simulink model "ACDCACsummarycircuit"  (R2023b)
settings: Solver=ode8  StartTime=0.0  StopTime=1  FixedStep=1e-7  MaxStep=1e-8  RelTol=1e-3
libraries: spsMosfetLib x6, spsSeriesRLCBranchLib x5, spsVoltageMeasurementLib x3, spsCurrentMeasurementLib x2, spsIGBTDiodeLib x2, powerlib_extras x2, spsTHDLib x2, simulink x2, spsACVoltageSourceLib x1, spsMeanLib x1, slpidlib x1, spsPLLLib x1
settings Model: SimulationMode=accelerator  Creator=LENOVO  LastModifiedBy=45276
settings SolverCC: ZeroCrossAlgorithm=Adaptive
settings DebuggingCC: MaskedZcDiagnostic=none  IgnoredZcDiagnostic=none

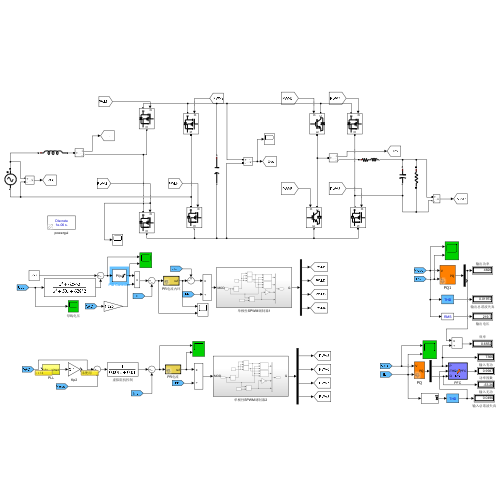
[thumbnail: Simulink's stored preview of the top-level diagram]
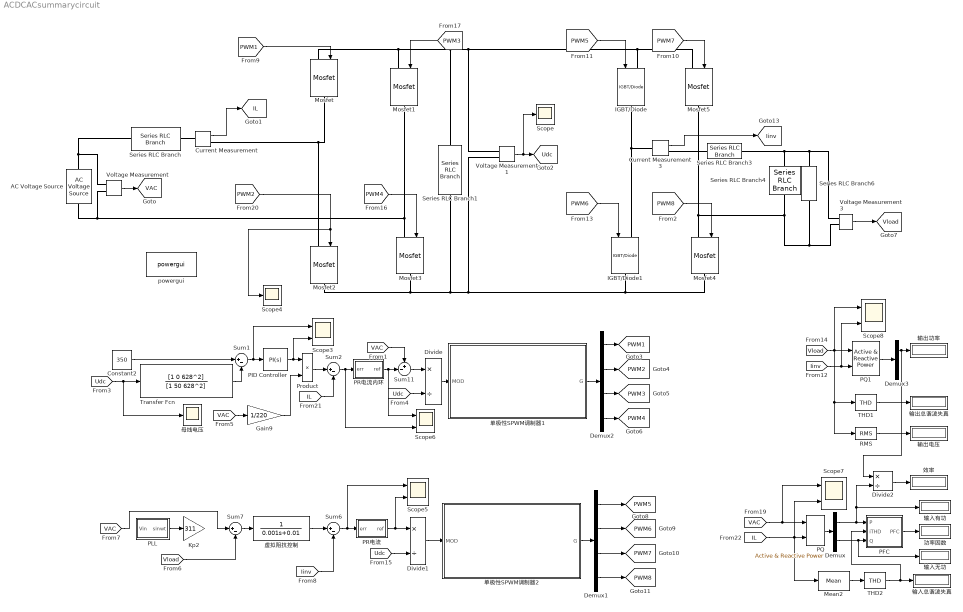
== system ACDCACsummarycircuit ==
  AC Voltage Source : spsACVoltageSourceLib/AC Voltage Source  Amplitude=311  Phase=0  Frequency=50  SampleTime=0  Measurements=None  BusType=swing  Pref=10e3  Qref=0  Qmin=-inf  Qmax=+inf
  Constant2 : Constant  Value=350
  Current Measurement : spsCurrentMeasurementLib/Current Measurement  PhasorSimulation=off  OutputType=Complex  PSBequivalent=0
  Current Measurement3 : spsCurrentMeasurementLib/Current Measurement  PhasorSimulation=off  OutputType=Complex  PSBequivalent=0
  Demux : Demux  Outputs=2
  Demux1 : Demux
  Demux2 : Demux
  Demux3 : Demux  Outputs=2
  Divide : Product  Inputs=*/
  Divide1 : Product  Inputs=*/
  Divide2 : Product  Inputs=*/
  Gain9 : Gain  Gain=1/220
  IGBT/Diode : spsIGBTDiodeLib/IGBT//Diode  Ron=1e-3  Rs=1e5  Cs=inf  Measurements=off
  IGBT/Diode1 : spsIGBTDiodeLib/IGBT//Diode  Ron=1e-3  Rs=1e5  Cs=inf  Measurements=off
  Kp2 : Gain  Gain=311
  Mean2 : spsMeanLib/Mean  Freq=10000  Vinit=0  Ts=0
  Mosfet{,1..5} (6 alike) : spsMosfetLib/Mosfet  Ron=0.05  Lon=0  Rd=0.01  Vfd=1  IC=0  Rs=1e5  Cs=inf  Measurements=off
  PFC : MATLAB Function  TreatAsAtomicUnit=on
  PID Controller : slpidlib/PID Controller  Controller=PI  Form=Parallel  TimeDomain=Continuous-time  UseExternalTs=off  SampleTime=-1  IntegratorMethod=Forward Euler  FilterMethod=Forward Euler  ControllerParametersSource=internal  P=0.4  I=10  UseKiTs=off  D=0.001  N=100  UseFilter=on  TunerSelectOption=Transfer Function Based (PID Tuner App)  InitialConditionSource=internal  InitialConditionForIntegrator=0  InitialConditionForFilter=0  DifferentiatorICPrevScaledInput=0  ExternalReset=none  TrackingMode=off  Kt=1  LimitOutput=on  SatLimitsSource=internal  UpperSaturationLimit=200  LowerSaturationLimit=-200  LinearizeAsGain=on  AntiWindupMode=clamping  Kb=1  LimitIntegrator=off  UpperIntegratorSaturationLimit=inf  LowerIntegratorSaturationLimit=-inf  POutMin=[]  POutMax=[]  IOutMin=[]  IOutMax=[]  DOutMin=[]  DOutMax=[]  NOutMin=[]  NOutMax=[]  SumOutMin=[]  SumOutMax=[]  SaturationOutMin=[]  SaturationOutMax=[]  PParamMin=[]  PParamMax=[]  IParamMin=[]  IParamMax=[]  DParamMin=[]  DParamMax=[]  NParamMin=[]  NParamMax=[]  KbParamMin=[]  KbParamMax=[]  KtParamMin=[]  KtParamMax=[]  KbOutMin=[]  KbOutMax=[]  KtOutMin=[]  KtOutMax=[]  IntegratorOutMin=[]  IntegratorOutMax=[]  FilterOutMin=[]  FilterOutMax=[]  SumI1OutMin=[]  SumI1OutMax=[]  SumI2OutMin=[]  SumI2OutMax=[]  SumI3OutMin=[]  SumI3OutMax=[]  SumI4OutMin=[]  SumI4OutMax=[]  SumDOutMin=[]  SumDOutMax=[]  DifferentiatorOutMin=[]  DifferentiatorOutMax=[]  FilterDiffOutCoefMin=[]  FilterDiffOutCoefMax=[]  ReciprocalOutMin=[]  ReciprocalOutMax=[]  SumDenOutMin=[]  SumDenOutMax=[]  SumNumOutMin=[]  SumNumOutMax=[]  DivideOutMin=[]  DivideOutMax=[]  UdiffTsProdOutMin=[]  UdiffTsProdOutMax=[]  NTsProdOutMin=[]  NTsProdOutMax=[]  UintegralTsProdOutMin=[]  UintegralTsProdOutMax=[]  UngainTsProdOutMin=[]  UngainTsProdOutMax=[]  ClampingZeroOutDataTypeStr=Inherit: Inherit via back propagation  ClampingZeroOutMin=[]  ClampingZeroOutMax=[]  FilterDenConstantOutDataTypeStr=Inherit: Inherit via back propagation  FilterDenConstantOutMin=[]  FilterDenConstantOutMax=[]  PCopyOutDataTypeStr=Inherit: Inherit via back propagation  PCopyOutMin=[]  PCopyOutMax=[]  NCopyOutDataTypeStr=Inherit: Inherit via back propagation  NCopyOutMin=[]  NCopyOutMax=[]  IntegratorContinuousStateAttributes=''  IntegratorStateMustResolveToSignalObject=off  IntegratorRTWStateStorageClass=Auto  FilterContinuousStateAttributes=''  FilterStateMustResolveToSignalObject=off  FilterRTWStateStorageClass=Auto  ParallelPVariant=InternalParameters  IdealPVariant=Disabled  IVariant=InternalParameters  DVariant=Disabled  IntegratorVariant=Continuous  SatVariant=Enabled  AWVariant=ContClampingParallel  PCopyVariant=Disabled  TRVariant=Disabled  FdbkBlocksVariant=Forward  IdealPFdbkVariant=Disabled  SatFdbkVariant=Disabled  DerivativeFilterVariant=Disabled  NVariant=Disabled  NCopyVariant=Disabled_SignalSpec  FilterICVariant=Disabled  IntegratorICVariant=InternalICs  ExternalResetVariant=Disabled  TRSumVariant=Passthrough  SumFdbkVariant=Disabled  SumVariant=Sum_PI  TsampFilterVariant=InternalTs  TsampNgainVariant=Passthrough  TsampIntegralVariant=Disabled_SignalSpec  ExternalSaturationOutDataTypeStr=Inherit: Same as second input
  PLL : Subsystem
  PQ : powerlib_extras/Measurements/Active & Reactive Power  f1=50
  PQ1 : powerlib_extras/Measurements/Active & Reactive Power  f1=50
  PR电流 : Subsystem  TreatAsAtomicUnit=on  mask{Kp=2, Kr=300, Wc=5, Upper=1000, Lower=-1000}
  PR电流内环 : Subsystem  TreatAsAtomicUnit=on  mask{Kp=3, Kr=100, Wc=5, Upper=310, Lower=-310}
  Product : Product
  RMS : spsRMSLib/RMS  TrueRMS=on  Freq=50  RMSInit=200  Ts=0
  Scope : Scope
  Scope{3,5..8} (5 alike) : Scope  NumInputPorts=2
  Scope4 : Scope
  Series RLC Branch : spsSeriesRLCBranchLib/Series RLC Branch  LConnTagsString=__new0  RConnTagsString=__new0  BranchType=L  Resistance=1  Inductance=6e-4  SetiL0=off  InitialCurrent=0  Capacitance=1e-6  Setx0=off  InitialVoltage=0  Measurements=None
  Series RLC Branch1 : spsSeriesRLCBranchLib/Series RLC Branch  LConnTagsString=__new0  RConnTagsString=__new0  BranchType=C  Resistance=1  Inductance=1e-3  SetiL0=off  InitialCurrent=0  Capacitance=4e-3  Setx0=on  InitialVoltage=310  Measurements=None
  Series RLC Branch3 : spsSeriesRLCBranchLib/Series RLC Branch  LConnTagsString=__new0  RConnTagsString=__new0  BranchType=RL  Resistance=0.05  Inductance=1e-3  SetiL0=off  InitialCurrent=0  Capacitance=1e-6  Setx0=off  InitialVoltage=0  Measurements=None
  Series RLC Branch4 : spsSeriesRLCBranchLib/Series RLC Branch  LConnTagsString=__new0  RConnTagsString=__new0  BranchType=C  Resistance=0.0042  Inductance=1e-3  SetiL0=off  InitialCurrent=0  Capacitance=6e-6  Setx0=off  InitialVoltage=0  Measurements=None
  Series RLC Branch6 : spsSeriesRLCBranchLib/Series RLC Branch  LConnTagsString=__new0  RConnTagsString=__new0  BranchType=R  Resistance=10  Inductance=1e-3  SetiL0=off  InitialCurrent=0  Capacitance=1e-4  Setx0=off  InitialVoltage=0  Measurements=None
  Sum{1..2,6..7} (4 alike) : Sum  Inputs=|+-
  Sum11 : Sum  Inputs=+-|
  THD1 : spsTHDLib/THD  Freq=50  Ts=0
  THD2 : spsTHDLib/THD  Freq=50  Ts=0
  Transfer Fcn : TransferFcn  Numerator=[1 0 628^2]  Denominator=[1 50 628^2]
  Voltage Measurement : spsVoltageMeasurementLib/Voltage Measurement  PhasorSimulation=off  OutputType=Complex  PSBequivalent=0
  Voltage Measurement1 : spsVoltageMeasurementLib/Voltage Measurement  PhasorSimulation=off  OutputType=Complex  PSBequivalent=0
  Voltage Measurement3 : spsVoltageMeasurementLib/Voltage Measurement  PhasorSimulation=off  OutputType=Complex  PSBequivalent=0
  powergui : sps_lib/powergui  Priority=1  SimulationMode=Discrete  SampleTime=1e-6  frequency=60  Iterations=50  frequencyindice=50  Pbase=100e6  ErrMax=1e-4  UnitsV=kV  UnitsW=MW  buscounter=0  FunctionMessages=off  echomessages=off  EnableUseOfTLC=off  CurrentSourceSwitches=off  DisableSnubberDevices=off  DisableRonSwitches=off  DisableVfSwitches=off  DisplayEquations=off  AutomaticDiscreteSolvers=off  SolverType=Tustin/Backward Euler (TBE)  Interpol=off  ExternalGateDelay=off  methode=off  Ts=100  x0status=blocks  SPID=on  SwTol=0  HookPort=off  NonlinearTolerance=1e-4  nMaxIteration=100  ContinueOnMaxIteration=off  RestoreLinks=warning  ResistiveCurrentMeasurement=off  Frange=[0:2:500]  Ylog=off  Xlog=on  ShowGrid=off  save=off  variable=ZData  structure=0  ZoomFFT=off  StartTime=0.0  cycles=1  DisplayStyle=1  fundamental=60  FreqAxis=off  MaxFrequency=1000  frequencyindicesteady=1  RmsSteady=1  display=off
  功率因数 : Display
  单极性SPWM调制器1 : Subsystem
  单极性SPWM调制器2 : Subsystem
  效率 : Display
  母线电压 : Scope
  虚拟阻抗控制 : TransferFcn  Numerator=1  Denominator=[0.001 0.01]
  输入总谐波失真 : Display
  输入无功 : Display
  输入有功 : Display
  输出功率 : Display
  输出总谐波失真 : Display
  输出电压 : Display
  tag scope: IL=global, Iinv=global, PWM1=global, PWM2=global, PWM3=global, PWM4=global, PWM5=global, PWM6=global, PWM7=global, PWM8=global, Udc=global, VAC=global, Vload=global
  wires:
  Voltage Measurement3/1 -> [Vload]
  [PWM6] -> IGBT/Diode1/1
  [PWM5] -> IGBT/Diode/1
  Current Measurement3/1 -> [Iinv]
  [PWM1] -> Mosfet/1
  [PWM2] -> Scope4/1, Mosfet2/1
  Voltage Measurement/1 -> [VAC]
  Current Measurement/1 -> [IL]
  Constant2/1 -> Sum1/1
  Sum1/1 -> Scope3/1, PID Controller/1
  Gain9/1 -> Product/2
  PID Controller/1 -> Scope3/2, Product/1
  Product/1 -> Sum2/1
  Transfer Fcn/1 -> Sum1/2
  Sum2/1 -> Scope6/2, PR电流内环/1(err)
  [IL] -> Sum2/2
  [Udc] -> Transfer Fcn/1, 母线电压/1
  PR电流内环/1(ref) -> Scope6/1, Sum11/2
  [VAC] -> Sum11/1
  Sum11/1 -> Divide/1
  [Udc] -> Divide/2
  [VAC] -> Gain9/1
  Demux2/1 -> [PWM1]
  Demux2/2 -> [PWM2]
  Sum7/1 -> 虚拟阻抗控制/1
  [Iinv] -> Sum6/2
  [Vload] -> Sum7/2
  PLL/1(sinwt) -> Kp2/1
  虚拟阻抗控制/1 -> Sum6/1
  PR电流/1(ref) -> Scope5/2, Divide1/1
  Sum6/1 -> Scope5/1, PR电流/1(err)
  Divide1/1 -> 单极性SPWM调制器2/1(MOD)
  [Udc] -> Divide1/2
  [PWM4] -> Mosfet3/1
  [PWM3] -> Mosfet1/1
  Divide/1 -> 单极性SPWM调制器1/1(MOD)
  单极性SPWM调制器1/1(G) -> Demux2/1
  Voltage Measurement1/1 -> Scope/1, [Udc]
  Demux/2 -> 输入无功/1, PFC/3(Q)
  THD2/1 -> 输入总谐波失真/1, PFC/2(iTHD)
  THD1/1 -> 输出总谐波失真/1
  Mean2/1 -> THD2/1
  Demux/1 -> Divide2/2, 输入有功/1, PFC/1(P)
  PQ/1 -> Demux/1
  [Vload] -> Scope8/1, RMS/1, THD1/1, PQ1/1
  RMS/1 -> 输出电压/1
  Demux3/1 -> Divide2/1, 输出功率/1
  Divide2/1 -> 效率/1
  PQ1/1 -> Demux3/1
  [VAC] -> PQ/1, Scope7/1
  [IL] -> Mean2/1, PQ/2, Scope7/2
  [Iinv] -> Scope8/2, PQ1/2
  PFC/1(PFC) -> 功率因数/1
  Demux2/3 -> [PWM3]
  Demux2/4 -> [PWM4]
  [PWM8] -> Mosfet4/1
  [PWM7] -> Mosfet5/1
  Demux1/4 -> [PWM8]
  Demux1/3 -> [PWM7]
  单极性SPWM调制器2/1(G) -> Demux1/1
  Demux1/2 -> [PWM6]
  Demux1/1 -> [PWM5]
  [VAC] -> Sum7/1
  connections:
  Voltage Measurement/LConn2 -- Mosfet1/RConn1 -- Mosfet3/LConn1 -- AC Voltage Source/LConn1
  Voltage Measurement3/LConn1 -- Series RLC Branch6/LConn1 -- Series RLC Branch3/RConn1 -- Series RLC Branch4/LConn1
  IGBT/Diode/RConn1 -- IGBT/Diode1/LConn1 -- Current Measurement3/LConn1
  Current Measurement3/RConn1 -- Series RLC Branch3/LConn1
  IGBT/Diode1/RConn1 -- Voltage Measurement1/LConn2 -- Series RLC Branch1/RConn1 -- Mosfet3/RConn1 -- Mosfet2/RConn1 -- Mosfet4/RConn1
  AC Voltage Source/RConn1 -- Voltage Measurement/LConn1 -- Series RLC Branch/LConn1
  Voltage Measurement1/LConn1 -- Mosfet5/LConn1 -- IGBT/Diode/LConn1 -- Series RLC Branch1/LConn1 -- Mosfet1/LConn1 -- Mosfet/LConn1
  Mosfet/RConn1 -- Mosfet2/LConn1 -- Current Measurement/RConn1
  Current Measurement/LConn1 -- Series RLC Branch/RConn1
  Mosfet4/LConn1 -- Mosfet5/RConn1 -- Series RLC Branch6/RConn1 -- Voltage Measurement3/LConn2 -- Series RLC Branch4/RConn1

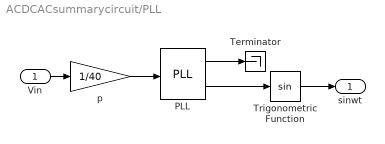
== system ACDCACsummarycircuit/PLL ==
  Vin : Inport
  PLL : spsPLLLib/PLL  Fmin=45  Par_Init=[0, 50]  ParK=[180, 3200, 1]  TcD=1e-4  MaxRateChangeFreq=12  FilterCutOffFreq=25  Ts=0  AGC=on
  Terminator : Terminator
  Trigonometric Function : Trigonometry
  p : Gain  Gain=1/40
  sinwt : Outport
  wires:
  PLL/2 -> Trigonometric Function/1
  PLL/1 -> Terminator/1
  p/1 -> PLL/1
  Trigonometric Function/1 -> sinwt/1
  Vin/1 -> p/1

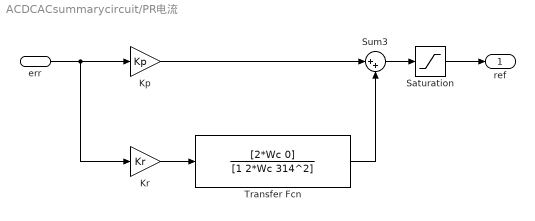
== system ACDCACsummarycircuit/PR电流 ==
  err : Inport
  Kp : Gain  Gain=Kp
  Kr : Gain  Gain=Kr
  Saturation : Saturate  UpperLimit=Upper  LowerLimit=Lower
  Sum3 : Sum  Inputs=|++
  Transfer Fcn : TransferFcn  Numerator=[2*Wc 0]  Denominator=[1 2*Wc 314^2]
  ref : Outport
  wires:
  Kp/1 -> Sum3/1
  Sum3/1 -> Saturation/1
  err/1 -> Kr/1, Kp/1
  Kr/1 -> Transfer Fcn/1
  Transfer Fcn/1 -> Sum3/2
  Saturation/1 -> ref/1

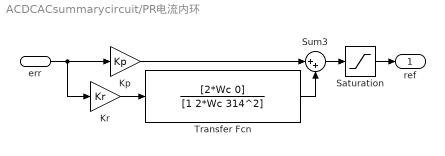
== system ACDCACsummarycircuit/PR电流内环 ==
  err : Inport
  Kp : Gain  Gain=Kp
  Kr : Gain  Gain=Kr
  Saturation : Saturate  UpperLimit=Upper  LowerLimit=Lower
  Sum3 : Sum  Inputs=|++
  Transfer Fcn : TransferFcn  Numerator=[2*Wc 0]  Denominator=[1 2*Wc 314^2]
  ref : Outport
  wires:
  Kp/1 -> Sum3/1
  Kr/1 -> Transfer Fcn/1
  Transfer Fcn/1 -> Sum3/2
  Saturation/1 -> ref/1
  err/1 -> Kr/1, Kp/1
  Sum3/1 -> Saturation/1

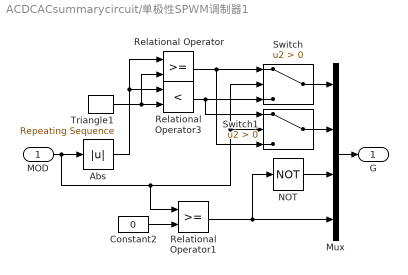
== system ACDCACsummarycircuit/单极性SPWM调制器1 ==
  MOD : Inport
  Abs : Abs  SaturateOnIntegerOverflow=off
  Constant2 : Constant  Value=0
  Mux : Mux
  NOT : Logic  Operator=NOT  IconShape=distinctive  AllPortsSameDT=off  OutDataTypeStr=boolean
  Relational Operator : RelationalOperator  OutDataTypeStr=boolean  InputSameDT=off
  Relational Operator1 : RelationalOperator  OutDataTypeStr=boolean  InputSameDT=off
  Relational Operator3 : RelationalOperator  Operator=<  OutDataTypeStr=boolean  InputSameDT=off
  Switch : Switch  Criteria=u2 > Threshold  SaturateOnIntegerOverflow=off  InputSameDT=off
  Switch1 : Switch  Criteria=u2 > Threshold  SaturateOnIntegerOverflow=off  InputSameDT=off
  Triangle1 : simulink/Sources/Repeating Sequence  rep_seq_t=[0 1/20000/2 1/20000]  rep_seq_y=[0 1 0]
  G : Outport
  wires:
  NOT/1 -> Mux/3
  Constant2/1 -> Relational Operator1/2
  Relational Operator1/1 -> NOT/1, Mux/4
  Abs/1 -> Relational Operator3/1, Relational Operator/1
  MOD/1 -> Abs/1, Relational Operator1/1, Switch/2, Switch1/2
  Mux/1 -> G/1
  Triangle1/1 -> Relational Operator3/2, Relational Operator/2
  Relational Operator/1 -> Switch1/3, Switch/1
  Switch/1 -> Mux/1
  Switch1/1 -> Mux/2
  Relational Operator3/1 -> Switch/3, Switch1/1

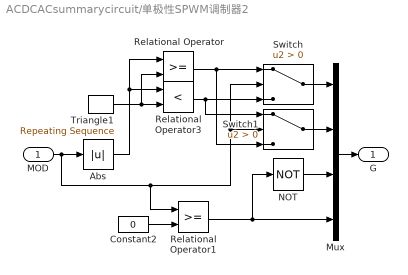
== system ACDCACsummarycircuit/单极性SPWM调制器2 ==
  MOD : Inport
  Abs : Abs  SaturateOnIntegerOverflow=off
  Constant2 : Constant  Value=0
  Mux : Mux
  NOT : Logic  Operator=NOT  IconShape=distinctive  AllPortsSameDT=off  OutDataTypeStr=boolean
  Relational Operator : RelationalOperator  OutDataTypeStr=boolean  InputSameDT=off
  Relational Operator1 : RelationalOperator  OutDataTypeStr=boolean  InputSameDT=off
  Relational Operator3 : RelationalOperator  Operator=<  OutDataTypeStr=boolean  InputSameDT=off
  Switch : Switch  Criteria=u2 > Threshold  SaturateOnIntegerOverflow=off  InputSameDT=off
  Switch1 : Switch  Criteria=u2 > Threshold  SaturateOnIntegerOverflow=off  InputSameDT=off
  Triangle1 : simulink/Sources/Repeating Sequence  rep_seq_t=[0 1/20000/2 1/20000]  rep_seq_y=[0 1 0]
  G : Outport
  wires:
  Relational Operator3/1 -> Switch1/1, Switch/3
  Switch1/1 -> Mux/2
  Switch/1 -> Mux/1
  Relational Operator/1 -> Switch/1, Switch1/3
  Triangle1/1 -> Relational Operator/2, Relational Operator3/2
  Mux/1 -> G/1
  MOD/1 -> Switch1/2, Switch/2, Relational Operator1/1, Abs/1
  Abs/1 -> Relational Operator/1, Relational Operator3/1
  Relational Operator1/1 -> Mux/4, NOT/1
  Constant2/1 -> Relational Operator1/2
  NOT/1 -> Mux/3

== matlab function ACDCACsummarycircuit/PFC ==
  data: P input; iTHD input; PFC output; Q input
function PFC = fcn(P,iTHD,Q)
% This block supports an embeddable subset of the MATLAB language.
% See the help menu for details. 
PFC=(P/sqrt(P*P+Q*Q))/sqrt(1+iTHD*iTHD);
